simulink model "simulink_model"  (R2013b)
settings: Solver=ode45  StartTime=0.0  StopTime=30  RelTol=1e-3
settings Model: Creator=petter  LastModifiedBy=petter

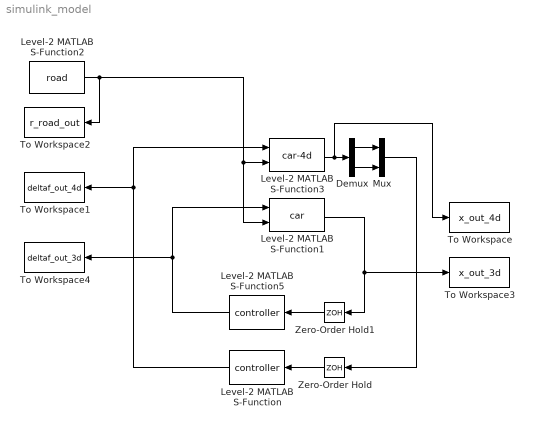
== system simulink_model ==
  Demux : Demux  Outputs=[1 1 2]
  Level-2 MATLAB S-Function : M-S-Function  FunctionName=controller  Parameters=1
  Level-2 MATLAB S-Function1 : M-S-Function  FunctionName=car
  Level-2 MATLAB S-Function2 : M-S-Function  FunctionName=road
  Level-2 MATLAB S-Function3 : M-S-Function  FunctionName=car-4d
  Level-2 MATLAB S-Function5 : M-S-Function  FunctionName=controller  Parameters=1
  Mux : Mux  Inputs=2
  To Workspace : ToWorkspace  VariableName=x_out_4d  SampleTime=-1  SaveFormat=Structure With Time
  To Workspace1 : ToWorkspace  VariableName=deltaf_out_4d  SampleTime=-1  SaveFormat=Structure With Time
  To Workspace2 : ToWorkspace  VariableName=r_road_out  SampleTime=-1  SaveFormat=Structure With Time
  To Workspace3 : ToWorkspace  VariableName=x_out_3d  SampleTime=-1  SaveFormat=Structure With Time
  To Workspace4 : ToWorkspace  VariableName=deltaf_out_3d  SampleTime=-1  SaveFormat=Structure With Time
  Zero-Order Hold : ZeroOrderHold  SampleTime=0.05
  Zero-Order Hold1 : ZeroOrderHold  SampleTime=0.05
  wires:
  Level-2 MATLAB S-Function/1 -> Level-2 MATLAB S-Function3/1, To Workspace1/1
  Level-2 MATLAB S-Function2/1 -> Level-2 MATLAB S-Function3/2, Level-2 MATLAB S-Function1/2, To Workspace2/1
  Zero-Order Hold/1 -> Level-2 MATLAB S-Function/1
  Level-2 MATLAB S-Function3/1 -> To Workspace/1, Demux/1
  Demux/1 -> Mux/1
  Demux/3 -> Mux/2
  Level-2 MATLAB S-Function1/1 -> Zero-Order Hold1/1, To Workspace3/1
  Mux/1 -> Zero-Order Hold/1
  Level-2 MATLAB S-Function5/1 -> To Workspace4/1, Level-2 MATLAB S-Function1/1
  Zero-Order Hold1/1 -> Level-2 MATLAB S-Function5/1
